simulink model "slrt_mat_playback"  (R2023b)
settings: Solver=FixedStepDiscrete  StartTime=0.0  StopTime=12  FixedStep=0.001  RelTol=1e-3
undefined symbols (not defined in the file or in its folder): replay_left_torque_bp, replay_left_torque_data, replay_phi_bp, replay_phi_data, replay_right_torque_bp, replay_right_torque_data
libraries: slrealtimeloglib x4
settings Model: Creator=Administrator  LastModifiedBy=Administrator
settings SolverCC: ConcurrentTasks=on  PositivePriorityOrder=on
settings OptimizationCC: BlockReduction=off  OptimizeBlockIOStorage=off
settings DebuggingCC: TasksWithSamePriorityMsg=none
settings HardwareCC: ProdBitPerLong=64  ProdLongLongMode=on  ProdHWDeviceType=Intel->x86-64 (Linux 64)
settings RTWCC: Description=Simulink Real-Time  SystemTargetFile=slrealtime.tlc  TemplateMakefile=slrealtime_default_tmf  Toolchain=Simulink Real-Time Toolchain  BuildConfiguration=Faster Runs  CodeExecutionProfiling=on  TargetLang=C++
settings SimulinkRealTimeTargetCC: SLRTFileLogMaxRuns=5

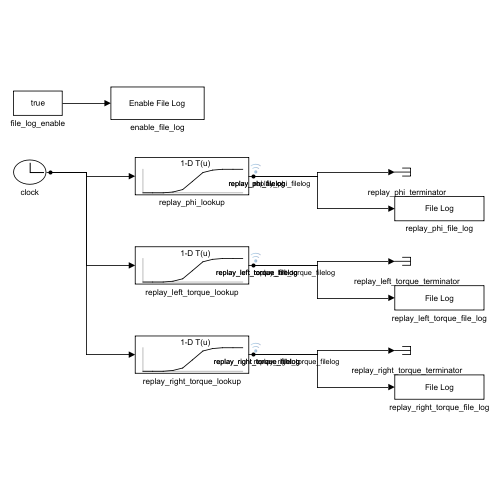
[thumbnail: Simulink's stored preview of the top-level diagram]
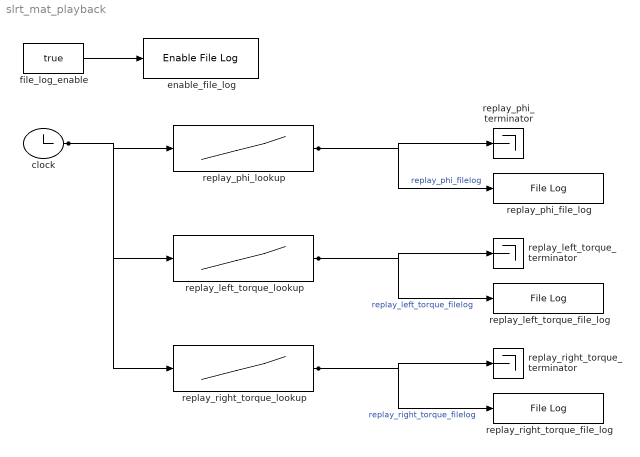
== system slrt_mat_playback ==
  clock : Clock
  enable_file_log : slrealtimeloglib/Enable File Log
  file_log_enable : Constant  Value=true  OutDataTypeStr=boolean
  replay_left_torque_file_log : slrealtimeloglib/File Log  decimation=10  inputProcessing=Elements as channels (sample based)
  replay_left_torque_lookup : Lookup_n-D  NumberOfTableDimensions=1  BreakpointsForDimension1=replay_left_torque_bp  Table=replay_left_torque_data  ExtrapMethod=Clip  InternalRulePriority=Speed  RndMeth=Simplest
  replay_left_torque_terminator : Terminator
  replay_phi_file_log : slrealtimeloglib/File Log  decimation=10  inputProcessing=Elements as channels (sample based)
  replay_phi_lookup : Lookup_n-D  NumberOfTableDimensions=1  BreakpointsForDimension1=replay_phi_bp  Table=replay_phi_data  ExtrapMethod=Clip  InternalRulePriority=Speed  RndMeth=Simplest
  replay_phi_terminator : Terminator
  replay_right_torque_file_log : slrealtimeloglib/File Log  decimation=10  inputProcessing=Elements as channels (sample based)
  replay_right_torque_lookup : Lookup_n-D  NumberOfTableDimensions=1  BreakpointsForDimension1=replay_right_torque_bp  Table=replay_right_torque_data  ExtrapMethod=Clip  InternalRulePriority=Speed  RndMeth=Simplest
  replay_right_torque_terminator : Terminator
  wires:
  file_log_enable/1 -> enable_file_log/1
  clock/1 -> replay_phi_lookup/1, replay_left_torque_lookup/1, replay_right_torque_lookup/1
  replay_phi_lookup/1 -> replay_phi_terminator/1, replay_phi_file_log/1  "replay_phi_filelog"
  replay_left_torque_lookup/1 -> replay_left_torque_terminator/1, replay_left_torque_file_log/1  "replay_left_torque_filelog"
  replay_right_torque_lookup/1 -> replay_right_torque_terminator/1, replay_right_torque_file_log/1  "replay_right_torque_filelog"
